simulink model "Simulink_20_10"  (R2020a)
settings: Solver=VariableStepAuto  StartTime=0.0  StopTime=75  RelTol=1e-3
values from neighbouring files (symbols this model uses):
  K_LQR = Ks(:,[1:4])    [Script_LQR.m]    (also in Workspace_20_Octubre.mat = [7.44426617397 -3.57630651915 0.414882035318 -0.177478528659; Workspace_21_Octubre.mat = [49.0239916482 -5.91602934063 2.652370576 -0.0810790967812])
  K_REI = [Ks(:,1) Ks(:,2)]    [Retro_Alimentacion_Integral.m]    (also in Workspace_20_Octubre.mat = [18.874405068 -8.29205202847 -9.96547850829 -1.40770716274]; Workspace_21_Octubre.mat = [34.4760176193 -15.5235439726 -4.32287066177 -1.41201865408])
  Ki_LQR = -Ks(:,[5])    [Script_LQR.m]    (also in Workspace_20_Octubre.mat = 0.632455532034; Workspace_21_Octubre.mat = 20)
  Ki_REI = -Ks(:,3)    [Retro_Alimentacion_Integral.m]    (also in Workspace_20_Octubre.mat = 7.05565296496; Workspace_21_Octubre.mat = 13.3109774254)
undefined symbols (not defined in the file or in its folder): Kd_ms, Ki_ms, Kp_ms
libraries: cstblocks x6, simulink x3
settings Model: Creator=geral  LastModifiedBy=geral

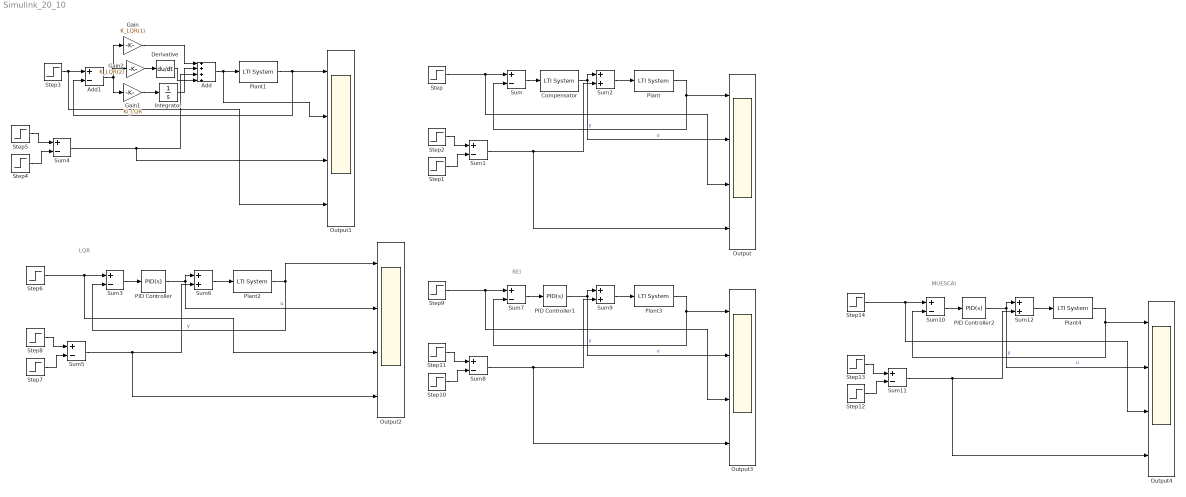
== system Simulink_20_10 ==
  note: REI
  note: LQR
  note: MUESCAI
  Add : Sum  Inputs=++++
  Add1 : Sum  Inputs=+-
  Compensator : cstblocks/LTI System  sys=C_IMC  IC=[]
  Derivative : Derivative
  Gain : Gain  Gain=K_LQR(1)
  Gain1 : Gain  Gain=Ki_LQR
  Gain2 : Gain  Gain=K_LQR(2)
  Integrator : Integrator
  Output{,1..4} (5 alike) : Scope  NumInputPorts=4
  PID Controller : simulink/Continuous/PID Controller  Controller=PID  Form=Parallel  TimeDomain=Continuous-time  UseExternalTs=off  SampleTime=-1  IntegratorMethod=Forward Euler  FilterMethod=Forward Euler  ControllerParametersSource=internal  P=K_LQR(1)  I=Ki_LQR  D=K_LQR(2)  UseFilter=on  N=15  TunerSelectOption=Transfer Function Based (PID Tuner App)  InitialConditionSource=internal  InitialConditionForIntegrator=0  InitialConditionForFilter=0  DifferentiatorICPrevScaledInput=0  ExternalReset=none  TrackingMode=off  Kt=1  LimitOutput=off  UpperSaturationLimit=inf  LowerSaturationLimit=-inf  LinearizeAsGain=on  AntiWindupMode=none  Kb=1  POutMin=[]  POutMax=[]  IOutMin=[]  IOutMax=[]  DOutMin=[]  DOutMax=[]  NOutMin=[]  NOutMax=[]  SumOutMin=[]  SumOutMax=[]  SaturationOutMin=[]  SaturationOutMax=[]  PParamMin=[]  PParamMax=[]  IParamMin=[]  IParamMax=[]  DParamMin=[]  DParamMax=[]  NParamMin=[]  NParamMax=[]  KbParamMin=[]  KbParamMax=[]  KtParamMin=[]  KtParamMax=[]  KbOutMin=[]  KbOutMax=[]  KtOutMin=[]  KtOutMax=[]  IntegratorOutMin=[]  IntegratorOutMax=[]  FilterOutMin=[]  FilterOutMax=[]  SumI1OutMin=[]  SumI1OutMax=[]  SumI2OutMin=[]  SumI2OutMax=[]  SumI3OutMin=[]  SumI3OutMax=[]  SumI4OutMin=[]  SumI4OutMax=[]  SumDOutMin=[]  SumDOutMax=[]  DifferentiatorOutMin=[]  DifferentiatorOutMax=[]  FilterDiffOutCoefMin=[]  FilterDiffOutCoefMax=[]  ReciprocalOutMin=[]  ReciprocalOutMax=[]  SumDenOutMin=[]  SumDenOutMax=[]  SumNumOutMin=[]  SumNumOutMax=[]  DivideOutMin=[]  DivideOutMax=[]  UdiffTsProdOutMin=[]  UdiffTsProdOutMax=[]  NTsProdOutMin=[]  NTsProdOutMax=[]  UintegralTsProdOutMin=[]  UintegralTsProdOutMax=[]  UngainTsProdOutMin=[]  UngainTsProdOutMax=[]  IntegratorContinuousStateAttributes=''  IntegratorStateMustResolveToSignalObject=off  IntegratorRTWStateStorageClass=Auto  FilterContinuousStateAttributes=''  FilterStateMustResolveToSignalObject=off  FilterRTWStateStorageClass=Auto  ParallelPVariant=InternalParameters  IdealPVariant=Disabled  IVariant=InternalParameters  DVariant=InternalParameters  IntegratorVariant=Continuous  SatVariant=Disabled  AWVariant=Passthrough  PCopyVariant=Disabled  TRVariant=Disabled  FdbkBlocksVariant=Forward  IdealPFdbkVariant=Disabled  SatFdbkVariant=Disabled  DerivativeFilterVariant=ContFilter  NVariant=InternalParameters  NCopyVariant=Disabled  FilterICVariant=InternalICsFilter  IntegratorICVariant=InternalICs  ExternalResetVariant=Disabled  TRSumVariant=Passthrough  SumFdbkVariant=Disabled  SumVariant=Sum_PID  TsampFilterVariant=InternalTs  TsampNgainVariant=Passthrough  TsampIntegralVariant=Passthrough
  PID Controller1 : simulink/Continuous/PID Controller  Controller=PID  Form=Parallel  TimeDomain=Continuous-time  UseExternalTs=off  SampleTime=-1  IntegratorMethod=Forward Euler  FilterMethod=Forward Euler  ControllerParametersSource=internal  P=K_REI(1)/7  I=Ki_REI/7  D=K_REI(2)/7  UseFilter=on  N=20  TunerSelectOption=Transfer Function Based (PID Tuner App)  InitialConditionSource=internal  InitialConditionForIntegrator=0  InitialConditionForFilter=0  DifferentiatorICPrevScaledInput=0  ExternalReset=none  TrackingMode=off  Kt=1  LimitOutput=off  UpperSaturationLimit=inf  LowerSaturationLimit=-inf  LinearizeAsGain=on  AntiWindupMode=none  Kb=1  POutMin=[]  POutMax=[]  IOutMin=[]  IOutMax=[]  DOutMin=[]  DOutMax=[]  NOutMin=[]  NOutMax=[]  SumOutMin=[]  SumOutMax=[]  SaturationOutMin=[]  SaturationOutMax=[]  PParamMin=[]  PParamMax=[]  IParamMin=[]  IParamMax=[]  DParamMin=[]  DParamMax=[]  NParamMin=[]  NParamMax=[]  KbParamMin=[]  KbParamMax=[]  KtParamMin=[]  KtParamMax=[]  KbOutMin=[]  KbOutMax=[]  KtOutMin=[]  KtOutMax=[]  IntegratorOutMin=[]  IntegratorOutMax=[]  FilterOutMin=[]  FilterOutMax=[]  SumI1OutMin=[]  SumI1OutMax=[]  SumI2OutMin=[]  SumI2OutMax=[]  SumI3OutMin=[]  SumI3OutMax=[]  SumI4OutMin=[]  SumI4OutMax=[]  SumDOutMin=[]  SumDOutMax=[]  DifferentiatorOutMin=[]  DifferentiatorOutMax=[]  FilterDiffOutCoefMin=[]  FilterDiffOutCoefMax=[]  ReciprocalOutMin=[]  ReciprocalOutMax=[]  SumDenOutMin=[]  SumDenOutMax=[]  SumNumOutMin=[]  SumNumOutMax=[]  DivideOutMin=[]  DivideOutMax=[]  UdiffTsProdOutMin=[]  UdiffTsProdOutMax=[]  NTsProdOutMin=[]  NTsProdOutMax=[]  UintegralTsProdOutMin=[]  UintegralTsProdOutMax=[]  UngainTsProdOutMin=[]  UngainTsProdOutMax=[]  IntegratorContinuousStateAttributes=''  IntegratorStateMustResolveToSignalObject=off  IntegratorRTWStateStorageClass=Auto  FilterContinuousStateAttributes=''  FilterStateMustResolveToSignalObject=off  FilterRTWStateStorageClass=Auto  ParallelPVariant=InternalParameters  IdealPVariant=Disabled  IVariant=InternalParameters  DVariant=InternalParameters  IntegratorVariant=Continuous  SatVariant=Disabled  AWVariant=Passthrough  PCopyVariant=Disabled  TRVariant=Disabled  FdbkBlocksVariant=Forward  IdealPFdbkVariant=Disabled  SatFdbkVariant=Disabled  DerivativeFilterVariant=ContFilter  NVariant=InternalParameters  NCopyVariant=Disabled  FilterICVariant=InternalICsFilter  IntegratorICVariant=InternalICs  ExternalResetVariant=Disabled  TRSumVariant=Passthrough  SumFdbkVariant=Disabled  SumVariant=Sum_PID  TsampFilterVariant=InternalTs  TsampNgainVariant=Passthrough  TsampIntegralVariant=Passthrough
  PID Controller2 : simulink/Continuous/PID Controller  Controller=PID  Form=Parallel  TimeDomain=Continuous-time  UseExternalTs=off  SampleTime=-1  IntegratorMethod=Forward Euler  FilterMethod=Forward Euler  ControllerParametersSource=internal  P=Kp_ms  I=Ki_ms  D=Kd_ms  UseFilter=on  N=30  TunerSelectOption=Transfer Function Based (PID Tuner App)  InitialConditionSource=internal  InitialConditionForIntegrator=0  InitialConditionForFilter=0  DifferentiatorICPrevScaledInput=0  ExternalReset=none  TrackingMode=off  Kt=1  LimitOutput=off  UpperSaturationLimit=inf  LowerSaturationLimit=-inf  LinearizeAsGain=on  AntiWindupMode=none  Kb=1  POutMin=[]  POutMax=[]  IOutMin=[]  IOutMax=[]  DOutMin=[]  DOutMax=[]  NOutMin=[]  NOutMax=[]  SumOutMin=[]  SumOutMax=[]  SaturationOutMin=[]  SaturationOutMax=[]  PParamMin=[]  PParamMax=[]  IParamMin=[]  IParamMax=[]  DParamMin=[]  DParamMax=[]  NParamMin=[]  NParamMax=[]  KbParamMin=[]  KbParamMax=[]  KtParamMin=[]  KtParamMax=[]  KbOutMin=[]  KbOutMax=[]  KtOutMin=[]  KtOutMax=[]  IntegratorOutMin=[]  IntegratorOutMax=[]  FilterOutMin=[]  FilterOutMax=[]  SumI1OutMin=[]  SumI1OutMax=[]  SumI2OutMin=[]  SumI2OutMax=[]  SumI3OutMin=[]  SumI3OutMax=[]  SumI4OutMin=[]  SumI4OutMax=[]  SumDOutMin=[]  SumDOutMax=[]  DifferentiatorOutMin=[]  DifferentiatorOutMax=[]  FilterDiffOutCoefMin=[]  FilterDiffOutCoefMax=[]  ReciprocalOutMin=[]  ReciprocalOutMax=[]  SumDenOutMin=[]  SumDenOutMax=[]  SumNumOutMin=[]  SumNumOutMax=[]  DivideOutMin=[]  DivideOutMax=[]  UdiffTsProdOutMin=[]  UdiffTsProdOutMax=[]  NTsProdOutMin=[]  NTsProdOutMax=[]  UintegralTsProdOutMin=[]  UintegralTsProdOutMax=[]  UngainTsProdOutMin=[]  UngainTsProdOutMax=[]  IntegratorContinuousStateAttributes=''  IntegratorStateMustResolveToSignalObject=off  IntegratorRTWStateStorageClass=Auto  FilterContinuousStateAttributes=''  FilterStateMustResolveToSignalObject=off  FilterRTWStateStorageClass=Auto  ParallelPVariant=InternalParameters  IdealPVariant=Disabled  IVariant=InternalParameters  DVariant=InternalParameters  IntegratorVariant=Continuous  SatVariant=Disabled  AWVariant=Passthrough  PCopyVariant=Disabled  TRVariant=Disabled  FdbkBlocksVariant=Forward  IdealPFdbkVariant=Disabled  SatFdbkVariant=Disabled  DerivativeFilterVariant=ContFilter  NVariant=InternalParameters  NCopyVariant=Disabled  FilterICVariant=InternalICsFilter  IntegratorICVariant=InternalICs  ExternalResetVariant=Disabled  TRSumVariant=Passthrough  SumFdbkVariant=Disabled  SumVariant=Sum_PID  TsampFilterVariant=InternalTs  TsampNgainVariant=Passthrough  TsampIntegralVariant=Passthrough
  Plant{,1..4} (5 alike) : cstblocks/LTI System  sys=tf10  IC=[]
  Step{,3,6,9,14} (5 alike) : Step  Time=0.1  After=0.7  SampleTime=0
  Step1 : Step  Time=25  After=0.1  SampleTime=0
  Step10 : Step  Time=40  After=0.1  SampleTime=0
  Step{4,8,11,13} (4 alike) : Step  Time=35  After=0.1  SampleTime=0
  Step12 : Step  Time=40  After=0.1  SampleTime=0
  Step2 : Step  Time=20  After=0.1  SampleTime=0
  Step5 : Step  Time=30  After=0.1  SampleTime=0
  Step7 : Step  Time=40  After=0.1  SampleTime=0
  Sum{,1,3..5,7..8,10..11} (9 alike) : Sum  Inputs=+-
  Sum{2,6,9,12} (4 alike) : Sum
  wires:
  Sum/1 -> Compensator/1
  Plant/1 -> Sum/2, Output/1  "y"
  Step/1 -> Output/3, Sum/1
  Step2/1 -> Sum1/1
  Step1/1 -> Sum1/2
  Sum2/1 -> Plant/1
  Compensator/1 -> Output/2, Sum2/1  "u"
  Sum1/1 -> Output/4, Sum2/2
  Step4/1 -> Sum4/2
  Step5/1 -> Sum4/1
  Plant1/1 -> Add1/2, Output1/1
  Gain1/1 -> Integrator/1
  Add/1 -> Output1/2, Plant1/1
  Integrator/1 -> Add/2
  Gain/1 -> Add/1
  Step3/1 -> Output1/4, Add1/1
  Add1/1 -> Gain1/1, Gain2/1, Gain/1
  Sum4/1 -> Output1/3, Add/3
  Gain2/1 -> Derivative/1
  Derivative/1 -> Add/4
  Step8/1 -> Sum5/1
  Sum6/1 -> Plant2/1
  Sum5/1 -> Output2/4, Sum6/2
  Plant2/1 -> Sum3/2, Output2/1  "y"
  PID Controller/1 -> Output2/2, Sum6/1  "u"
  Step6/1 -> Output2/3, Sum3/1
  Step7/1 -> Sum5/2
  Sum3/1 -> PID Controller/1
  PID Controller1/1 -> Output3/2, Sum9/1  "u"
  Sum7/1 -> PID Controller1/1
  Sum9/1 -> Plant3/1
  Step11/1 -> Sum8/1
  Step9/1 -> Output3/3, Sum7/1
  Plant3/1 -> Sum7/2, Output3/1  "y"
  Sum8/1 -> Output3/4, Sum9/2
  Step10/1 -> Sum8/2
  Sum11/1 -> Output4/4, Sum12/2
  Step12/1 -> Sum11/2
  Plant4/1 -> Sum10/2, Output4/1  "y"
  PID Controller2/1 -> Output4/2, Sum12/1  "u"
  Sum10/1 -> PID Controller2/1
  Step13/1 -> Sum11/1
  Step14/1 -> Output4/3, Sum10/1
  Sum12/1 -> Plant4/1
